simulink model "VDSE_2019b"  (R2025b)
settings: Solver=ode5  StartTime=0.0  StopTime=inf  FixedStep=simulation_step_time  RelTol=1e-3
values from neighbouring files (symbols this model uses):
  A = 1    [vehicle_parameters_script.m]
  bump_height = 0    [vehicle_parameters_script.m]
  bump_length = 1    [vehicle_parameters_script.m]
  bump_time = 1    [vehicle_parameters_script.m]
  cd = 1.8    [vehicle_parameters_script.m]
  cF = 1000    [vehicle_parameters_script.m]
  clF = -cl*(1-Aero_balance)    (= 1.344)    [vehicle_parameters_script.m]
  clR = -cl*Aero_balance    (= 1.456)    [vehicle_parameters_script.m]
  cp_FA = 30    [vehicle_parameters_script.m]
  cp_RA = 13    [vehicle_parameters_script.m]
  cR = 1000    [vehicle_parameters_script.m]
  ctF = tireF.VERTICAL_DAMPING    [vehicle_parameters_script.m]
  ctR = tireR.VERTICAL_DAMPING    [vehicle_parameters_script.m]
  enableAWD = 1    [vehicle_parameters_script.m]
  enableLongDynamics = 1    [vehicle_parameters_script.m]
  enablePowertrain = 1    [vehicle_parameters_script.m]
  Engine_Speed = readmatrix('EngineMap.xlsx','Range','B2:B20')    [vehicle_parameters_script.m]
  Engine_Torque = readmatrix('EngineMap.xlsx','Range','A2:A20')    [vehicle_parameters_script.m]
  exf = 10e-12    (= 1e-11)    [Paceijka52_Parameters.m]
  exr = 10e-12    (= 1e-11)    [Paceijka52_Parameters.m]
  eyf = 1e-12    [Paceijka52_Parameters.m]
  eyr = 1e-12    [Paceijka52_Parameters.m]
  FNOMINf = tireF.FNOMIN    [Paceijka52_Parameters.m]
  FNOMINr = tireR.FNOMIN    [Paceijka52_Parameters.m]
  g = 9.806    [vehicle_parameters_script.m]
  GR = 5.3    [vehicle_parameters_script.m]
  hcog = 0.3054    [vehicle_parameters_script.m]
  hpc = 0.0    (= 0)    [vehicle_parameters_script.m]
  hrcF = 0    [vehicle_parameters_script.m]
  hrcg = (hrcF*lR+hrcR*lF)/(lF+lR)    (= 0)    [vehicle_parameters_script.m]
  hrcR = 0    [vehicle_parameters_script.m]
  huFcog = 0.3054    [vehicle_parameters_script.m]
  huRcog = 0.3054    [vehicle_parameters_script.m]
  JwF = 0.32    [vehicle_parameters_script.m]
  JwR = 0.32    [vehicle_parameters_script.m]
  Jx = 73    [vehicle_parameters_script.m]
  Jy = 230    [vehicle_parameters_script.m]
  Jz = 220    [vehicle_parameters_script.m]
  kF = 40000    [vehicle_parameters_script.m]
  kR = 35000    [vehicle_parameters_script.m]
  kRF = 0    [vehicle_parameters_script.m]
  kRR = 0    [vehicle_parameters_script.m]
  ktF = tireF.VERTICAL_STIFFNESS    [vehicle_parameters_script.m]
  ktR = tireR.VERTICAL_STIFFNESS    [vehicle_parameters_script.m]
  lF = 1.223    [vehicle_parameters_script.m]
  lR = l-lF    (= 0.307)    [vehicle_parameters_script.m]
  m = 258.612    [vehicle_parameters_script.m]
  max_pressure = 1000    [vehicle_parameters_script.m]
  mF = 10.347    [vehicle_parameters_script.m]
  mR = 10.347    [vehicle_parameters_script.m]
  PCX1f = tireF.PCX1    [Paceijka52_Parameters.m]
  PCX1r = tireR.PCX1    [Paceijka52_Parameters.m]
  PCY1f = tireF.PCY1    [Paceijka52_Parameters.m]
  PCY1r = tireR.PCY1    [Paceijka52_Parameters.m]
  PDX1f = tireF.PDX1    [Paceijka52_Parameters.m]
  PDX1r = tireR.PDX1    [Paceijka52_Parameters.m]
  PDX2f = tireF.PDX2    [Paceijka52_Parameters.m]
  PDX2r = tireR.PDX2    [Paceijka52_Parameters.m]
  PDY1f = tireF.PDY1    [Paceijka52_Parameters.m]
  PDY1r = tireR.PDY1    [Paceijka52_Parameters.m]
  PDY2f = tireF.PDY2    [Paceijka52_Parameters.m]
  PDY2r = tireR.PDY2    [Paceijka52_Parameters.m]
  PDY3f = tireF.PDY3    [Paceijka52_Parameters.m]
  PDY3r = tireR.PDY3    [Paceijka52_Parameters.m]
  PEX1f = tireF.PEX1    [Paceijka52_Parameters.m]
  PEX1r = tireR.PEX1    [Paceijka52_Parameters.m]
  PEX2f = tireF.PEX2    [Paceijka52_Parameters.m]
  PEX2r = tireR.PEX2    [Paceijka52_Parameters.m]
  PEX3f = tireF.PEX3    [Paceijka52_Parameters.m]
  PEX3r = tireR.PEX3    [Paceijka52_Parameters.m]
  PEX4f = tireF.PEX4    [Paceijka52_Parameters.m]
  PEX4r = tireR.PEX4    [Paceijka52_Parameters.m]
  PEY1f = tireF.PEY1    [Paceijka52_Parameters.m]
  PEY1r = tireR.PEY1    [Paceijka52_Parameters.m]
  PEY2f = tireF.PEY2    [Paceijka52_Parameters.m]
  PEY2r = tireR.PEY2    [Paceijka52_Parameters.m]
  PEY3f = tireF.PEY3    [Paceijka52_Parameters.m]
  PEY3r = tireR.PEY3    [Paceijka52_Parameters.m]
  PEY4f = tireF.PEY4    [Paceijka52_Parameters.m]
  PEY4r = tireR.PEY4    [Paceijka52_Parameters.m]
  phi0 = 0    [vehicle_parameters_script.m]
  phi_dot0 = 0    [vehicle_parameters_script.m]
  PHX1f = tireF.PHX1    [Paceijka52_Parameters.m]
  PHX1r = tireR.PHX1    [Paceijka52_Parameters.m]
  PHX2f = tireF.PHX2    [Paceijka52_Parameters.m]
  PHX2r = tireR.PHX2    [Paceijka52_Parameters.m]
  PHY1f = tireF.PHY1    [Paceijka52_Parameters.m]
  PHY1r = tireR.PHY1    [Paceijka52_Parameters.m]
  PHY2f = tireF.PHY2    [Paceijka52_Parameters.m]
  PHY2r = tireR.PHY2    [Paceijka52_Parameters.m]
  PHY3f = tireF.PHY3    [Paceijka52_Parameters.m]
  PHY3r = tireR.PHY3    [Paceijka52_Parameters.m]
  PKX1f = tireF.PKX1    [Paceijka52_Parameters.m]
  PKX1r = tireR.PKX1    [Paceijka52_Parameters.m]
  PKX2f = tireF.PKX2    [Paceijka52_Parameters.m]
  PKX2r = tireR.PKX2    [Paceijka52_Parameters.m]
  PKX3f = tireF.PKX3    [Paceijka52_Parameters.m]
  PKX3r = tireR.PKX3    [Paceijka52_Parameters.m]
  PKY1f = tireF.PKY1    [Paceijka52_Parameters.m]
  PKY1r = tireR.PKY1    [Paceijka52_Parameters.m]
  PKY2f = tireF.PKY2    [Paceijka52_Parameters.m]
  PKY2r = tireR.PKY2    [Paceijka52_Parameters.m]
  PKY3f = tireF.PKY3    [Paceijka52_Parameters.m]
  PKY3r = tireR.PKY3    [Paceijka52_Parameters.m]
  psi0 = 0    [vehicle_parameters_script.m]
  psi_dot0 = 0    [vehicle_parameters_script.m]
  PVX1f = tireF.PVX1    [Paceijka52_Parameters.m]
  PVX1r = tireR.PVX1    [Paceijka52_Parameters.m]
  PVX2f = tireF.PVX2    [Paceijka52_Parameters.m]
  PVX2r = tireR.PVX2    [Paceijka52_Parameters.m]
  PVY1f = tireF.PVY1    [Paceijka52_Parameters.m]
  PVY1r = tireR.PVY1    [Paceijka52_Parameters.m]
  PVY2f = tireF.PVY2    [Paceijka52_Parameters.m]
  PVY2r = tireR.PVY2    [Paceijka52_Parameters.m]
  PVY3f = tireF.PVY3    [Paceijka52_Parameters.m]
  PVY3r = tireR.PVY3    [Paceijka52_Parameters.m]
  PVY4f = tireF.PVY4    [Paceijka52_Parameters.m]
  PVY4r = tireR.PVY4    [Paceijka52_Parameters.m]
  QBZ10f = tireF.QBZ10    [Paceijka52_Parameters.m]
  QBZ10r = tireR.QBZ10    [Paceijka52_Parameters.m]
  ... (+143 more)
undefined symbols (not defined in the file or in its folder): Bxf, Bxr, Byf, Byr, Cxf, Cxr, Cyf, Cyr, Dxf, Dxr, Dyf, Dyr, FFB_Gain
libraries: mfeval_LIB x4, sim3dlib x1, sim3dautolib x1, sl3dlib x1
(part 3 of 5)

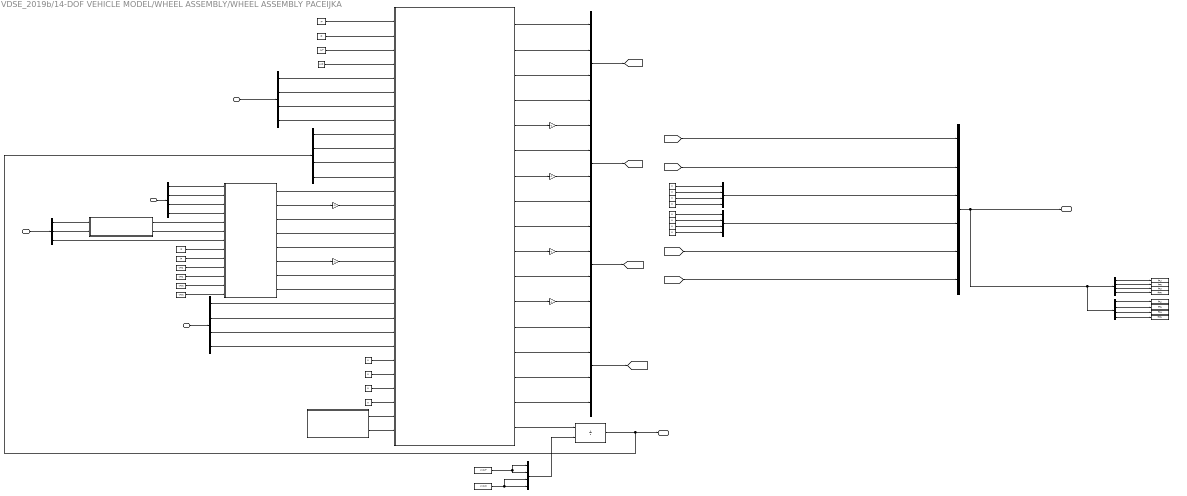
== system VDSE_2019b/14-DOF VEHICLE MODEL/WHEEL ASSEMBLY/WHEEL ASSEMBLY PACEIJKA ==
  note: EXPORTING TIRE FORCES AND MOMENTS
  note: SAVING TIRE FORCES
  steer input [rad] : Inport
  sprung mass outputs : Inport  Port=2
  unsprung masses outputs : Inport  Port=3
  Torques [Nm] : Inport  Port=4
  Bus Creator : BusCreator  Inputs=6
  Bus Creator{1..4,7..8} (6 alike) : BusCreator  Inputs=4
  Bus Selector : BusSelector  OutputSignals=Unsprung masses z Forces [N].FLz_Overall [N],Unsprung masses z Forces [N].FRz_Overall [N],Unsprung masses z Forces [N].RLz_Overall [N],Unsprung masses z Forces [N].RRz_Overall [N]
  Bus Selector2 : BusSelector  OutputSignals=Longitudinal Dynamics.Vx [m/s],Lateral Dynamics.Vy [m/s],Yaw dynamics.psi_dot [rad/s]
  Bus Selector3 : BusSelector  OutputSignals=Steering.deltaFL [rad],Steering.deltaFR [rad],Steering.deltaRL [rad],Steering.deltaRR [rad]
  Bus Selector5 : BusSelector  OutputSignals=TFL [Nm],TFR [Nm],TRL [Nm],TRR [Nm]
  Bus Selector6 : BusSelector  OutputSignals=Tyre x Forces [N].fFLx [N],Tyre x Forces [N].fFRx [N],Tyre x Forces [N].fRLx [N],Tyre x Forces [N].fRRx [N]
  Bus Selector7 : BusSelector  OutputSignals=Tyre y Forces [N].fFLy [N],Tyre y Forces [N].fFRy [N],Tyre y Forces [N].fRLy [N],Tyre y Forces [N].fRRy [N]
  Constant{,26..28} (4 alike) : Constant  Value=0
  Constant1 : Constant  Value=wF/2
  Constant13 : Constant  Value=lF
  Constant14 : Constant  Value=lR
  Constant2 : Constant  Value=wF/2
  Constant20 : Constant  Value=rF
  Constant21 : Constant  Value=rR
  Constant22 : Constant  Value=JwF
  Constant23 : Constant  Value=JwR
  Constant24 : Constant  Value=Vx0/rF
  Constant25 : Constant  Value=Vx0/rR
  Constant3 : Constant  Value=wR/2
  Constant4 : Constant  Value=wR/2
  Demux1 : Demux
  Gain{,1..5} (6 alike) : Gain  Gain=-1
  Integrator1 : Integrator  InitialConditionSource=external
  Mux2 : Mux
  SIDE SLIP ANGLE CALCULATION : Subsystem
  TIRE FORCES AND WHEEL DYNAMICS : MATLAB Function  TreatAsAtomicUnit=on
  TIRE PARAMETERS : Subsystem
  TIRE VELOCITIES : MATLAB Function  TreatAsAtomicUnit=on
  To Workspace : ToWorkspace  VariableName=fFLx  SaveFormat=Timeseries  SampleTime=-1
  To Workspace1 : ToWorkspace  VariableName=fFRx  SaveFormat=Timeseries  SampleTime=-1
  To Workspace2 : ToWorkspace  VariableName=fRLx  SaveFormat=Timeseries  SampleTime=-1
  To Workspace3 : ToWorkspace  VariableName=fRRx  SaveFormat=Timeseries  SampleTime=-1
  To Workspace4 : ToWorkspace  VariableName=fFLy  SaveFormat=Timeseries  SampleTime=-1
  To Workspace5 : ToWorkspace  VariableName=fFRy  SaveFormat=Timeseries  SampleTime=-1
  To Workspace6 : ToWorkspace  VariableName=fRLy  SaveFormat=Timeseries  SampleTime=-1
  To Workspace7 : ToWorkspace  VariableName=fRRy  SaveFormat=Timeseries  SampleTime=-1
  Zero{,1..7} (8 alike) : Constant  Value=0  OutDataTypeStr=Inherit: Inherit via back propagation
  Tyre Forces and Moments : Outport
  Wheel Speeds [rad/s] : Outport  Port=2
  wires:
  Zero/1 -> Bus Creator3/1  "fFLz [N]"
  Zero2/1 -> Bus Creator3/3  "fRLz [N]"
  Zero4/1 -> Bus Creator4/1  "mFLx [Nm]"
  Zero1/1 -> Bus Creator3/2  "fFRz [N]"
  Zero7/1 -> Bus Creator4/4  "mRRx [Nm]"
  Zero5/1 -> Bus Creator4/2  "mFRx [Nm]"
  Zero3/1 -> Bus Creator3/4  "fRRz [N]"
  Zero6/1 -> Bus Creator4/3  "mRLx [Nm]"
  Bus Creator2/1 -> [Tyre_y_Forces]  "Tyre y Forces [N]"
  TIRE FORCES AND WHEEL DYNAMICS/7(fRLy) -> Gain2/1  "fRLy [N]"
  TIRE FORCES AND WHEEL DYNAMICS/5(fFLy) -> Gain3/1  "fFLy [N]"
  Bus Creator1/1 -> [Tyre_x_Forces]  "Tyre x Forces [N]"
  TIRE VELOCITIES/8(VRRy) -> TIRE FORCES AND WHEEL DYNAMICS/20(VRRy)  "VRRy"
  TIRE VELOCITIES/7(VRRx) -> TIRE FORCES AND WHEEL DYNAMICS/19(VRRx)  "VRRx"
  Integrator1/1 -> Wheel Speeds [rad/s]/1, Demux1/1  "omega [rad/s]"
  Demux1/4 -> TIRE FORCES AND WHEEL DYNAMICS/12(omegaRR)
  Demux1/3 -> TIRE FORCES AND WHEEL DYNAMICS/11(omegaRL)
  Demux1/2 -> TIRE FORCES AND WHEEL DYNAMICS/10(omegaFR)
  Demux1/1 -> TIRE FORCES AND WHEEL DYNAMICS/9(omegaFL)
  TIRE FORCES AND WHEEL DYNAMICS/17(omega_dot) -> Integrator1/1  "omegas_dot [rad/s^2]"
  Constant25/1 -> Mux2/4, Mux2/3
  Mux2/1 -> Integrator1/2
  Constant24/1 -> Mux2/1, Mux2/2
  Constant21/1 -> TIRE FORCES AND WHEEL DYNAMICS/2(rR)
  Constant23/1 -> TIRE FORCES AND WHEEL DYNAMICS/4(JwR)
  Constant22/1 -> TIRE FORCES AND WHEEL DYNAMICS/3(JwF)
  Constant20/1 -> TIRE FORCES AND WHEEL DYNAMICS/1(rF)
  TIRE VELOCITIES/2(VFLy) -> Gain/1  "VFLy"
  TIRE VELOCITIES/1(VFLx) -> TIRE FORCES AND WHEEL DYNAMICS/13(VFLx)  "VFLx"
  TIRE VELOCITIES/4(VFRy) -> TIRE FORCES AND WHEEL DYNAMICS/16(VFRy)  "VFRy"
  Constant4/1 -> TIRE VELOCITIES/13(wRR)
  Constant13/1 -> TIRE VELOCITIES/8(lF)
  Constant1/1 -> TIRE VELOCITIES/10(wFL)
  Constant14/1 -> TIRE VELOCITIES/9(lR)
  Constant2/1 -> TIRE VELOCITIES/11(wFR)
  TIRE VELOCITIES/5(VRLx) -> TIRE FORCES AND WHEEL DYNAMICS/17(VRLx)  "VRLx"
  Constant3/1 -> TIRE VELOCITIES/12(wRL)
  TIRE VELOCITIES/3(VFRx) -> TIRE FORCES AND WHEEL DYNAMICS/15(VFRx)  "VFRx"
  TIRE VELOCITIES/6(VRLy) -> Gain1/1  "VRLy"
  SIDE SLIP ANGLE CALCULATION/2(beta [rad]) -> TIRE VELOCITIES/6(beta)  "beta"
  SIDE SLIP ANGLE CALCULATION/1(V [m/s]) -> TIRE VELOCITIES/5(V)  "V"
  Bus Selector/1 -> TIRE FORCES AND WHEEL DYNAMICS/5(fFLz)  "<FLz_Overall [N]>"
  Bus Selector/4 -> TIRE FORCES AND WHEEL DYNAMICS/8(fRRz)  "<RRz_Overall [N]>"
  Bus Selector/3 -> TIRE FORCES AND WHEEL DYNAMICS/7(fRLz)  "<RLz_Overall [N]>"
  Bus Selector/2 -> TIRE FORCES AND WHEEL DYNAMICS/6(fFRz)  "<FRz_Overall [N]>"
  unsprung masses outputs/1 -> Bus Selector/1
  sprung mass outputs/1 -> Bus Selector2/1
  Bus Selector3/2 -> TIRE VELOCITIES/2(deltaFR)  "<deltaFR [rad]>"
  Bus Selector3/4 -> TIRE VELOCITIES/4(deltaRR)  "<deltaRR [rad]>"
  Bus Selector3/1 -> TIRE VELOCITIES/1(deltaFL)  "<deltaFL [rad]>"
  Bus Selector3/3 -> TIRE VELOCITIES/3(deltaRL)  "<deltaRL [rad]>"
  steer input [rad]/1 -> Bus Selector3/1
  Bus Creator/1 -> Bus Selector7/1, Bus Selector6/1, Tyre Forces and Moments/1
  Torques [Nm]/1 -> Bus Selector5/1
  Bus Selector6/1 -> To Workspace/1  "<fFLx [N]>"
  Bus Selector6/2 -> To Workspace1/1  "<fFRx [N]>"
  Bus Selector6/3 -> To Workspace2/1  "<fRLx [N]>"
  Bus Selector6/4 -> To Workspace3/1  "<fRRx [N]>"
  Bus Selector7/1 -> To Workspace4/1  "<fFLy [N]>"
  Bus Selector7/2 -> To Workspace5/1  "<fFRy [N]>"
  Bus Selector7/3 -> To Workspace6/1  "<fRLy [N]>"
  Bus Selector7/4 -> To Workspace7/1  "<fRRy [N]>"
  [Tyre_y_Moments] -> Bus Creator/5  "Tyre My Moments [Nm]"
  Constant/1 -> TIRE FORCES AND WHEEL DYNAMICS/25(gammaFL)
  Constant26/1 -> TIRE FORCES AND WHEEL DYNAMICS/26(gammaFR)
  Constant27/1 -> TIRE FORCES AND WHEEL DYNAMICS/27(gammaRL)
  Constant28/1 -> TIRE FORCES AND WHEEL DYNAMICS/28(gammaRR)
  TIRE PARAMETERS/1(Tire Parameters Front Axle) -> TIRE FORCES AND WHEEL DYNAMICS/29(TireParams_front)
  TIRE PARAMETERS/2(Tire Parameters Rear Axle) -> TIRE FORCES AND WHEEL DYNAMICS/30(TireParams_rear)
  Gain/1 -> TIRE FORCES AND WHEEL DYNAMICS/14(VFLy)  "VFLy"
  Gain1/1 -> TIRE FORCES AND WHEEL DYNAMICS/18(VRLy)  "VRLy"
  TIRE FORCES AND WHEEL DYNAMICS/1(fFLx) -> Bus Creator1/1  "fFLx [N]"
  TIRE FORCES AND WHEEL DYNAMICS/2(fFRx) -> Bus Creator1/2  "fFRx [N]"
  TIRE FORCES AND WHEEL DYNAMICS/3(fRLx) -> Bus Creator1/3  "fRLx [N]"
  TIRE FORCES AND WHEEL DYNAMICS/4(fRRx) -> Bus Creator1/4  "fRRx [N]"
  Gain3/1 -> Bus Creator2/1  "fFLy [N]"
  TIRE FORCES AND WHEEL DYNAMICS/6(fFRy) -> Bus Creator2/2  "fFRy [N]"
  Gain2/1 -> Bus Creator2/3  "fRLy [N]"
  TIRE FORCES AND WHEEL DYNAMICS/8(fRRy) -> Bus Creator2/4  "fRRy [N]"
  [Tyre_x_Forces] -> Bus Creator/1  "Tyre x Forces [N]"
  [Tyre_y_Forces] -> Bus Creator/2  "Tyre y Forces [N]"
  Bus Creator3/1 -> Bus Creator/3  "Tyre z Forces [N]"
  Bus Creator4/1 -> Bus Creator/4  "Tyre Mx Moments [Nm]"
  [Tyre_z_Moments] -> Bus Creator/6  "Tyre Mz Moments [Nm]"
  TIRE FORCES AND WHEEL DYNAMICS/9(mFLz) -> Bus Creator7/1  "mFLz [Nm]"
  TIRE FORCES AND WHEEL DYNAMICS/10(mFRz) -> Gain4/1  "mFRz [Nm]"
  Gain4/1 -> Bus Creator7/2  "mFRz [Nm]"
  TIRE FORCES AND WHEEL DYNAMICS/11(mRLz) -> Bus Creator7/3  "mRLz [Nm]"
  TIRE FORCES AND WHEEL DYNAMICS/12(mRRz) -> Gain5/1  "mRRz [Nm]"
  Gain5/1 -> Bus Creator7/4  "mRRz [Nm]"
  TIRE FORCES AND WHEEL DYNAMICS/13(mFLy) -> Bus Creator8/1  "mFLy [Nm]"
  TIRE FORCES AND WHEEL DYNAMICS/14(mFRy) -> Bus Creator8/2  "mFRy [Nm]"
  TIRE FORCES AND WHEEL DYNAMICS/15(mRLy) -> Bus Creator8/3  "mRLy [Nm]"
  TIRE FORCES AND WHEEL DYNAMICS/16(mRRy) -> Bus Creator8/4  "mRRy [Nm]"
  Bus Creator7/1 -> [Tyre_z_Moments]  "Tyre Mz Moments [Nm]"
  Bus Creator8/1 -> [Tyre_y_Moments]  "Tyre My Moments [Nm]"
  Bus Selector2/1 -> SIDE SLIP ANGLE CALCULATION/1(Vx [m/s])  "<Vx [m/s]>"
  Bus Selector2/2 -> SIDE SLIP ANGLE CALCULATION/2(Vy [m/s])  "<Vy [m/s]>"
  Bus Selector2/3 -> TIRE VELOCITIES/7(psidot)  "<psi_dot [rad/s]>"
  Bus Selector5/1 -> TIRE FORCES AND WHEEL DYNAMICS/21(TFL)  "<TFL [Nm]>"
  Bus Selector5/2 -> TIRE FORCES AND WHEEL DYNAMICS/22(TFR)  "<TFR [Nm]>"
  Bus Selector5/3 -> TIRE FORCES AND WHEEL DYNAMICS/23(TRL)  "<TRL [Nm]>"
  Bus Selector5/4 -> TIRE FORCES AND WHEEL DYNAMICS/24(TRR)  "<TRR [Nm]>"

== system VDSE_2019b/14-DOF VEHICLE MODEL/EQUATIONS OF MOTION FOR CHASSIS/Pitch Dynamics/Downforce ==
  Vx : Inport
  Gain : Gain  Gain=-0.5*rho*clF*A
  Gain{1,3,5,7} (4 alike) : Gain  Gain=0.5
  Gain2 : Gain  Gain=-0.5*rho*clF*A
  Gain4 : Gain  Gain=-0.5*rho*clR*A
  Gain6 : Gain  Gain=-0.5*rho*clR*A
  Square{,1..3} (4 alike) : Math  Operator=square
  fFLz_overall : Outport
  fFRz_overall : Outport  Port=2
  fRLz_overall : Outport  Port=3
  fRRz_overall : Outport  Port=4
  wires:
  Gain/1 -> Gain1/1
  Square/1 -> Gain/1
  Gain1/1 -> fFLz_overall/1
  Square1/1 -> Gain2/1
  Gain2/1 -> Gain3/1
  Gain3/1 -> fFRz_overall/1
  Vx/1 -> Square/1, Square1/1, Square2/1, Square3/1
  Gain6/1 -> Gain7/1
  Square3/1 -> Gain6/1
  Square2/1 -> Gain4/1
  Gain4/1 -> Gain5/1
  Gain5/1 -> fRLz_overall/1
  Gain7/1 -> fRRz_overall/1

== system VDSE_2019b/14-DOF VEHICLE MODEL/EQUATIONS OF MOTION FOR CHASSIS/Roll Dynamics/Downforce ==
  Vx : Inport
  Gain : Gain  Gain=-0.5*rho*clF*A
  Gain{1,3,5,7} (4 alike) : Gain  Gain=0.5
  Gain2 : Gain  Gain=-0.5*rho*clF*A
  Gain4 : Gain  Gain=-0.5*rho*clR*A
  Gain6 : Gain  Gain=-0.5*rho*clR*A
  Square{,1..3} (4 alike) : Math  Operator=square
  fFLz_overall : Outport
  fFRz_overall : Outport  Port=2
  fRLz_overall : Outport  Port=3
  fRRz_overall : Outport  Port=4
  wires:
  Gain/1 -> Gain1/1
  Square/1 -> Gain/1
  Gain1/1 -> fFLz_overall/1
  Square1/1 -> Gain2/1
  Gain2/1 -> Gain3/1
  Gain3/1 -> fFRz_overall/1
  Vx/1 -> Square/1, Square1/1, Square2/1, Square3/1
  Gain6/1 -> Gain7/1
  Square3/1 -> Gain6/1
  Square2/1 -> Gain4/1
  Gain4/1 -> Gain5/1
  Gain5/1 -> fRLz_overall/1
  Gain7/1 -> fRRz_overall/1

== system VDSE_2019b/14-DOF VEHICLE MODEL/EQUATIONS OF MOTION FOR CHASSIS/Vertical Dynamics/Downforce ==
  Vx : Inport
  Gain : Gain  Gain=-0.5*rho*clF*A
  Gain{1,3,5,7} (4 alike) : Gain  Gain=0.5
  Gain2 : Gain  Gain=-0.5*rho*clF*A
  Gain4 : Gain  Gain=-0.5*rho*clR*A
  Gain6 : Gain  Gain=-0.5*rho*clR*A
  Square{,1..3} (4 alike) : Math  Operator=square
  fFLz_overall : Outport
  fFRz_overall : Outport  Port=2
  fRLz_overall : Outport  Port=3
  fRRz_overall : Outport  Port=4
  wires:
  Gain/1 -> Gain1/1
  Square/1 -> Gain/1
  Gain1/1 -> fFLz_overall/1
  Square1/1 -> Gain2/1
  Gain2/1 -> Gain3/1
  Gain3/1 -> fFRz_overall/1
  Vx/1 -> Square/1, Square1/1, Square2/1, Square3/1
  Gain6/1 -> Gain7/1
  Square3/1 -> Gain6/1
  Square2/1 -> Gain4/1
  Gain4/1 -> Gain5/1
  Gain5/1 -> fRLz_overall/1
  Gain7/1 -> fRRz_overall/1

== system VDSE_2019b/14-DOF VEHICLE MODEL/SUSPENSION/FRONT SUSPENSION/SUSPENSION FL ==
  z [m] : Inport
  Vz [m/s] : Inport  Port=2
  phi [rad] : Inport  Port=3
  phi_dot [rad/s] : Inport  Port=4
  theta [rad] : Inport  Port=5
  theta_dot [rad/s] : Inport  Port=6
  zFR [m] : Inport  Port=7
  yFL_road [m] : Inport  Port=8
  FL : Subsystem
  TIRE VERTICAL DEFLECTION : Subsystem
  fFLz [N] : Outport
  zFL_dot [m/s] : Outport  Port=2
  zFL [m] : Outport  Port=3
  wires:
  FL/2(zFL_dot [m/s]) -> TIRE VERTICAL DEFLECTION/2(zFL_dot [m/s]), zFL_dot [m/s]/1
  z [m]/1 -> FL/1(z [m])
  TIRE VERTICAL DEFLECTION/1(fFLz [N]) -> fFLz [N]/1
  theta [rad]/1 -> FL/5(theta [rad])
  zFR [m]/1 -> FL/7(zFR [m])
  Vz [m/s]/1 -> FL/2(Vz [m/s])
  yFL_road [m]/1 -> TIRE VERTICAL DEFLECTION/3(yFL_road [m]), FL/8(yFL_road [m])
  phi_dot [rad/s]/1 -> FL/4(phi_dot [rad/s])
  FL/1(zFL [m]) -> TIRE VERTICAL DEFLECTION/1(zFL [m]), zFL [m]/1
  phi [rad]/1 -> FL/3(phi [rad])
  theta_dot [rad/s]/1 -> FL/6(theta_dot [rad/s])

== system VDSE_2019b/14-DOF VEHICLE MODEL/SUSPENSION/FRONT SUSPENSION/SUSPENSION FR ==
  z [m] : Inport
  Vz [m/s] : Inport  Port=2
  phi [rad] : Inport  Port=3
  phi_dot [rad/s] : Inport  Port=4
  theta [rad] : Inport  Port=5
  theta_dot [rad/s] : Inport  Port=6
  zFL [m] : Inport  Port=7
  yFR_road [m] : Inport  Port=8
  FR : Subsystem
  TIRE VERTICAL DEFLECTION : Subsystem
  fFRz [N] : Outport
  zFR [m] : Outport  Port=2
  zFR_dot [m/s] : Outport  Port=3
  wires:
  FR/2(zFR_dot [m/s]) -> zFR_dot [m/s]/1, TIRE VERTICAL DEFLECTION/2(zFR_dot [m/s])
  yFR_road [m]/1 -> FR/8(yFR_road [m]), TIRE VERTICAL DEFLECTION/3(yFR_road [m])
  z [m]/1 -> FR/1(z [m])
  TIRE VERTICAL DEFLECTION/1(fFRz [N]) -> fFRz [N]/1
  theta [rad]/1 -> FR/5(theta [rad])
  zFL [m]/1 -> FR/7(zFL [m])
  Vz [m/s]/1 -> FR/2(Vz [m/s])
  phi_dot [rad/s]/1 -> FR/4(phi_dot [rad/s])
  FR/1(zFR [m]) -> TIRE VERTICAL DEFLECTION/1(zFR [m]), zFR [m]/1
  phi [rad]/1 -> FR/3(phi [rad])
  theta_dot [rad/s]/1 -> FR/6(theta_dot [rad/s])

== system VDSE_2019b/14-DOF VEHICLE MODEL/SUSPENSION/Load Transfer/Coupling of load transfer and suspension reaction ==
  Longidutinal Load Transfer [N] : Inport
  Lateral Load Transfer - Front [N] : Inport  Port=2
  Lateral Load Transfer - Rear [N] : Inport  Port=3
  <fFLz [N]> : Inport  Port=4
  <fFRz [N]> : Inport  Port=5
  <fRLz [N]> : Inport  Port=6
  <fRRz [N]> : Inport  Port=7
  Add{,1..4} (5 alike) : Sum
  Add5 : Sum  Inputs=+-
  Add6 : Sum  Inputs=-+
  Add7 : Sum  Inputs=--
  Lateral Load Transfer - Front [N]1 : InportShadow  Port=2
  Lateral Load Transfer - Rear [N]1 : InportShadow  Port=3
  Longidutinal Load Transfer [N]1 : InportShadow
  Longidutinal Load Transfer [N]2 : InportShadow
  Longidutinal Load Transfer [N]3 : InportShadow
  FLz_Overall [N] : Outport
  FRz_Overall [N] : Outport  Port=2
  RLz_Overall [N] : Outport  Port=3
  RRz_Overall [N] : Outport  Port=4
  wires:
  <fFRz [N]>/1 -> Add1/2
  Lateral Load Transfer - Rear [N]/1 -> Add5/2
  Longidutinal Load Transfer [N]/1 -> Add7/1
  Add7/1 -> Add/1  "FL Dynamic LT"
  Lateral Load Transfer - Front [N]/1 -> Add7/2
  Add4/1 -> Add3/1  "RR Dynamic LT"
  Add6/1 -> Add1/1  "FR Dynamic LT"
  Add5/1 -> Add2/1  "RL Dynamic LT"
  <fRRz [N]>/1 -> Add3/2
  <fFLz [N]>/1 -> Add/2
  <fRLz [N]>/1 -> Add2/2
  Add1/1 -> FRz_Overall [N]/1  "FRz_Overall [N]"
  Add3/1 -> RRz_Overall [N]/1  "RRz_Overall [N]"
  Add/1 -> FLz_Overall [N]/1  "FLz_Overall [N]"
  Add2/1 -> RLz_Overall [N]/1  "RLz_Overall [N]"
  Longidutinal Load Transfer [N]1/1 -> Add6/1
  Longidutinal Load Transfer [N]2/1 -> Add5/1
  Longidutinal Load Transfer [N]3/1 -> Add4/1
  Lateral Load Transfer - Front [N]1/1 -> Add6/2
  Lateral Load Transfer - Rear [N]1/1 -> Add4/2

== system VDSE_2019b/14-DOF VEHICLE MODEL/SUSPENSION/Load Transfer/Dynamic Lateral Load Transfer - Front ==
  ay [m/s^2] : Inport
  Add : Sum
  Gain : Gain  Gain=lR/(lR+lF)
  Gain1 : Gain  Gain=2*mF*huFcog/wF
  Gain2 : Gain  Gain=m*hrcF/wF
  Lat. Dynamic Transfer [N] : Outport
  wires:
  ay [m/s^2]/1 -> Gain2/1, Gain1/1
  Gain2/1 -> Gain/1
  Add/1 -> Lat. Dynamic Transfer [N]/1
  Gain1/1 -> Add/2
  Gain/1 -> Add/1

== system VDSE_2019b/14-DOF VEHICLE MODEL/SUSPENSION/Load Transfer/Dynamic Lateral Load Transfer - Rear ==
  ay [m/s^2] : Inport
  Add : Sum
  Gain : Gain  Gain=lF/(lR+lF)
  Gain1 : Gain  Gain=2*mR*huRcog/wR
  Gain2 : Gain  Gain=m*hrcR/wR
  Lat. Dynamic Transfer [N] : Outport
  wires:
  Add/1 -> Lat. Dynamic Transfer [N]/1
  Gain1/1 -> Add/2
  ay [m/s^2]/1 -> Gain2/1, Gain1/1
  Gain2/1 -> Gain/1
  Gain/1 -> Add/1

== system VDSE_2019b/14-DOF VEHICLE MODEL/SUSPENSION/Load Transfer/Dynamic Longitudinal Load Transfer ==
  ax [m/s^2] : Inport
  Add : Sum
  Gain : Gain  Gain=1/2*hpc*m/(lF+lR)/2
  Gain1 : Gain  Gain=(mF*huFcog + mR*huRcog)/(lF+lR)
  Long. Dynamic Transfer [N] : Outport
  wires:
  ax [m/s^2]/1 -> Gain1/1, Gain/1
  Gain/1 -> Add/1
  Add/1 -> Long. Dynamic Transfer [N]/1
  Gain1/1 -> Add/2

== system VDSE_2019b/14-DOF VEHICLE MODEL/SUSPENSION/REAR SUSPENSION/SUSPENSION RL ==
  z [m] : Inport
  Vz [m/s] : Inport  Port=2
  phi [rad] : Inport  Port=3
  phi_dot [rad/s] : Inport  Port=4
  theta [rad] : Inport  Port=5
  theta_dot [rad/s] : Inport  Port=6
  zRR [m] : Inport  Port=7
  yRL_road [m] : Inport  Port=8
  RL : Subsystem
  TIRE VERTICAL DEFLECTION : Subsystem
  fRLz [N] : Outport
  zRL_dot [m/s] : Outport  Port=2
  zRL [m] : Outport  Port=3
  wires:
  RL/2(zRL_dot [m/s]) -> TIRE VERTICAL DEFLECTION/2(zRL_dot [m/s]), zRL_dot [m/s]/1
  z [m]/1 -> RL/1(z [m])
  TIRE VERTICAL DEFLECTION/1(fRLz [N]) -> fRLz [N]/1  "fRLz [N]"
  theta [rad]/1 -> RL/5(theta [rad])
  zRR [m]/1 -> RL/7(zRR [m])
  Vz [m/s]/1 -> RL/2(Vz [m/s])
  yRL_road [m]/1 -> TIRE VERTICAL DEFLECTION/3(yRL_road [m]), RL/8(yRL_road [m])
  phi_dot [rad/s]/1 -> RL/4(phi_dot [rad/s])
  RL/1(zRL [m]) -> TIRE VERTICAL DEFLECTION/1(zRL [m]), zRL [m]/1
  phi [rad]/1 -> RL/3(phi [rad])
  theta_dot [rad/s]/1 -> RL/6(theta_dot [rad/s])

== system VDSE_2019b/14-DOF VEHICLE MODEL/SUSPENSION/REAR SUSPENSION/SUSPENSION RR ==
  z [m] : Inport
  Vz [m/s] : Inport  Port=2
  phi [rad] : Inport  Port=3
  phi_dot [rad/s] : Inport  Port=4
  theta [rad] : Inport  Port=5
  theta_dot [rad/s] : Inport  Port=6
  zRL [m] : Inport  Port=7
  yRR_road [m] : Inport  Port=8
  RR : Subsystem
  TIRE VERTICAL DEFLECTION : Subsystem
  fRRz [N] : Outport
  zRR [m] : Outport  Port=2
  zRR_dot [m/s] : Outport  Port=3
  wires:
  RR/2(zRR_dot [m/s]) -> TIRE VERTICAL DEFLECTION/2(zRR_dot [m/s]), zRR_dot [m/s]/1
  yRR_road [m]/1 -> TIRE VERTICAL DEFLECTION/3(yRR_road [m]), RR/8(yRR_road [m])
  z [m]/1 -> RR/1(z [m])
  TIRE VERTICAL DEFLECTION/1(fRRz [N]) -> fRRz [N]/1
  theta [rad]/1 -> RR/5(theta [rad])
  zRL [m]/1 -> RR/7(zRL [m])
  Vz [m/s]/1 -> RR/2(Vz [m/s])
  phi_dot [rad/s]/1 -> RR/4(phi_dot [rad/s])
  RR/1(zRR [m]) -> TIRE VERTICAL DEFLECTION/1(zRR [m]), zRR [m]/1
  phi [rad]/1 -> RR/3(phi [rad])
  theta_dot [rad/s]/1 -> RR/6(theta_dot [rad/s])

== system VDSE_2019b/14-DOF VEHICLE MODEL/WHEEL ASSEMBLY/WHEEL ASSEMBLY BCD/SIDE SLIP ANGLE CALCULATION ==
  Vx [m/s] : Inport
  Vy [m/s] : Inport  Port=2
  Add : Sum
  Atan2 : Trigonometry  Operator=atan2
  Clock : Clock
  Constant : Constant  Value=enableLongDynamics
  Constant1 : Constant  Value=Vx0
  Constant2 : Constant  Value=0
  Sqrt : Sqrt
  Square : Math  Operator=square
  Square1 : Math  Operator=square
  Switch : Switch  Criteria=u2 > Threshold  SaturateOnIntegerOverflow=off  InputSameDT=off
  Switch1 : Switch  Criteria=u2 > Threshold  Threshold=0.01  SaturateOnIntegerOverflow=off  InputSameDT=off
  Vy [m/s]1 : InportShadow  Port=2
  V [m/s] : Outport
  beta [rad] : Outport  Port=2
  wires:
  Clock/1 -> Switch1/2
  Constant2/1 -> Switch1/3
  Switch1/1 -> Switch/2
  Constant1/1 -> Switch/3
  Constant/1 -> Switch1/1
  Switch/1 -> Atan2/2, Square/1
  Square1/1 -> Add/2
  Square/1 -> Add/1
  Vy [m/s]/1 -> Square1/1
  Vx [m/s]/1 -> Switch/1
  Add/1 -> Sqrt/1
  Sqrt/1 -> V [m/s]/1
  Atan2/1 -> beta [rad]/1
  Vy [m/s]1/1 -> Atan2/1

== system VDSE_2019b/14-DOF VEHICLE MODEL/WHEEL ASSEMBLY/WHEEL ASSEMBLY BCD/TIRE PARAMETERS ==
  Constant : Constant  Value=Bxf
  Constant1 : Constant  Value=Cxf
  Constant10 : Constant  Value=Cyr
  Constant11 : Constant  Value=Dyr
  Constant2 : Constant  Value=Dxf
  Constant3 : Constant  Value=Bxr
  Constant4 : Constant  Value=Cxr
  Constant5 : Constant  Value=Dxr
  Constant6 : Constant  Value=Byf
  Constant7 : Constant  Value=Cyf
  Constant8 : Constant  Value=Dyf
  Constant9 : Constant  Value=Byr
  Bxf : Outport
  Cxf : Outport  Port=2
  Dxf : Outport  Port=3
  Bxr : Outport  Port=4
  Cxr : Outport  Port=5
  Dxr : Outport  Port=6
  Byf : Outport  Port=7
  Cyf : Outport  Port=8
  Dyf : Outport  Port=9
  Byr : Outport  Port=10
  Cyr : Outport  Port=11
  Dyr : Outport  Port=12
  wires:
  Constant/1 -> Bxf/1
  Constant1/1 -> Cxf/1
  Constant2/1 -> Dxf/1
  Constant5/1 -> Dxr/1
  Constant4/1 -> Cxr/1
  Constant3/1 -> Bxr/1
  Constant9/1 -> Byr/1
  Constant10/1 -> Cyr/1
  Constant11/1 -> Dyr/1
  Constant8/1 -> Dyf/1
  Constant7/1 -> Cyf/1
  Constant6/1 -> Byf/1

== system VDSE_2019b/14-DOF VEHICLE MODEL/WHEEL ASSEMBLY/WHEEL ASSEMBLY MFEVAL/SIDE SLIP ANGLE CALCULATION ==
  Vx [m/s] : Inport
  Vy [m/s] : Inport  Port=2
  Add : Sum
  Atan2 : Trigonometry  Operator=atan2
  Clock : Clock
  Constant : Constant  Value=enableLongDynamics
  Constant1 : Constant  Value=Vx0
  Constant2 : Constant  Value=0
  Sqrt : Sqrt
  Square : Math  Operator=square
  Square1 : Math  Operator=square
  Switch : Switch  Criteria=u2 > Threshold  SaturateOnIntegerOverflow=off  InputSameDT=off
  Switch1 : Switch  Criteria=u2 > Threshold  Threshold=0.01  SaturateOnIntegerOverflow=off  InputSameDT=off
  Vy [m/s]1 : InportShadow  Port=2
  V [m/s] : Outport
  beta [rad] : Outport  Port=2
  wires:
  Clock/1 -> Switch1/2
  Constant2/1 -> Switch1/3
  Switch1/1 -> Switch/2
  Constant1/1 -> Switch/3
  Constant/1 -> Switch1/1
  Square1/1 -> Add/2
  Square/1 -> Add/1
  Vy [m/s]/1 -> Square1/1
  Vx [m/s]/1 -> Switch/1
  Add/1 -> Sqrt/1
  Atan2/1 -> beta [rad]/1
  Vy [m/s]1/1 -> Atan2/1
  Switch/1 -> Atan2/2, Square/1
  Sqrt/1 -> V [m/s]/1

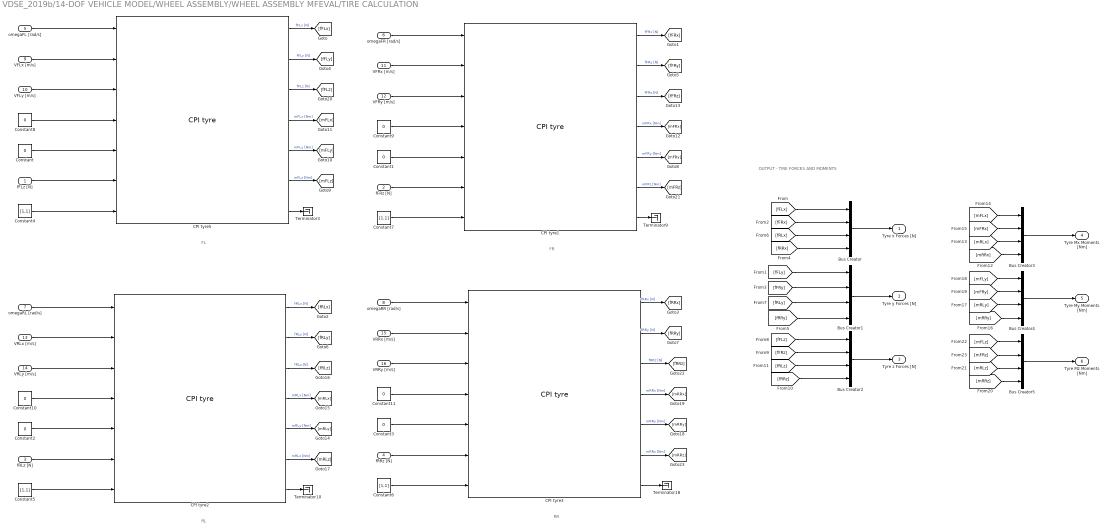
== system VDSE_2019b/14-DOF VEHICLE MODEL/WHEEL ASSEMBLY/WHEEL ASSEMBLY MFEVAL/TIRE CALCULATION ==
  note: RR
  note: RL
  note: FR
  note: FL
  note: OUTPUT - TIRE FORCES AND MOMENTS
  fFLz [N] : Inport
  fFRz [N] : Inport  Port=2
  fRLz [N] : Inport  Port=3
  fRRz [N] : Inport  Port=4
  omegaFL [rad/s] : Inport  Port=5
  omegaFR [rad/s] : Inport  Port=6
  omegaRL [rad/s] : Inport  Port=7
  omegaRR [rad/s] : Inport  Port=8
  VFLx [m/s] : Inport  Port=9
  VFLy [m/s] : Inport  Port=10
  VFRx [m/s] : Inport  Port=11
  VFRy [m/s] : Inport  Port=12
  VRLx [m/s] : Inport  Port=13
  VRLy [m/s] : Inport  Port=14
  VRRx [m/s] : Inport  Port=15
  VRRy [m/s] : Inport  Port=16
  Bus Creator{,1..5} (6 alike) : BusCreator  Inputs=4
  CPI tyre1 : mfeval_LIB/CPI tyre  Description=Magic Formula 6.1.2 tyre model including relaxation length and transient calculations  userParameterSource=tir_file_front  userSide=2 right  userDynamics=1 steady state  userUseMode=1 combined  enablePressure=off  userPressure=2.3
      settings: SourceProductName=MFeval Library
  CPI tyre2 : mfeval_LIB/CPI tyre  Description=Magic Formula 6.1.2 tyre model including relaxation length and transient calculations  userParameterSource=tir_file_rear  userSide=1 left  userDynamics=1 steady state  userUseMode=1 combined  enablePressure=off  userPressure=2.3
      settings: SourceProductName=MFeval Library
  CPI tyre3 : mfeval_LIB/CPI tyre  Description=Magic Formula 6.1.2 tyre model including relaxation length and transient calculations  userParameterSource=tir_file_rear  userSide=2 right  userDynamics=1 steady state  userUseMode=1 combined  enablePressure=off  userPressure=2.3
      settings: SourceProductName=MFeval Library
  CPI tyre5 : mfeval_LIB/CPI tyre  Description=Magic Formula 6.1.2 tyre model including relaxation length and transient calculations  userParameterSource=tir_file_front  userSide=1 left  userDynamics=1 steady state  userUseMode=1 combined  enablePressure=off  userPressure=2.3
      settings: SourceProductName=MFeval Library
  Constant{,1..3,8..11} (8 alike) : Constant  Value=0
  Constant{4..7} (4 alike) : Constant  Value=[1,1]
  Terminator{3,9..10,18} (4 alike) : Terminator
  Tyre x Forces [N] : Outport
  Tyre y Forces [N] : Outport  Port=2
  Tyre z Forces [N] : Outport  Port=3
  Tyre Mx Moments [Nm] : Outport  Port=4
  Tyre My Moments [Nm] : Outport  Port=5
  Tyre Mz Moments [Nm] : Outport  Port=6
  wires:
  Constant11/1 -> CPI tyre3/4
  Constant10/1 -> CPI tyre2/4
  Constant9/1 -> CPI tyre1/4
  Constant8/1 -> CPI tyre5/4
  CPI tyre3/3 -> [fRRz]  "fRRz [N]"
  CPI tyre3/6 -> [mRRz]  "mRRz [Nm]"
  CPI tyre3/4 -> [mRRx]  "mRRx [Nm]"
  CPI tyre3/5 -> [mRRy]  "mRRy [Nm]"
  CPI tyre2/3 -> [fRLz]  "fRLz [N]"
  CPI tyre2/6 -> [mRLz]  "mRLz [Nm]"
  CPI tyre2/4 -> [mRLx]  "mRLx [Nm]"
  CPI tyre2/5 -> [mRLy]  "mRLy [Nm]"
  CPI tyre1/3 -> [fFRz]  "fFRz [N]"
  CPI tyre1/6 -> [mFRz]  "mFRz [Nm]"
  CPI tyre1/4 -> [mFRx]  "mFRx [Nm]"
  CPI tyre1/5 -> [mFRy]  "mFRy [Nm]"
  CPI tyre5/3 -> [fFLz]  "fFLz [N]"
  CPI tyre5/4 -> [mFLx]  "mFLx [Nm]"
  CPI tyre5/5 -> [mFLy]  "mFLy [Nm]"
  Bus Creator5/1 -> Tyre Mz Moments [Nm]/1
  [mFRz] -> Bus Creator5/2
  [mRLz] -> Bus Creator5/3
  [mRRz] -> Bus Creator5/4
  [mFLz] -> Bus Creator5/1
  [mFLy] -> Bus Creator4/1
  [mRRy] -> Bus Creator4/4
  [mRLy] -> Bus Creator4/3
  [mFRy] -> Bus Creator4/2
  Bus Creator4/1 -> Tyre My Moments [Nm]/1
  Bus Creator3/1 -> Tyre Mx Moments [Nm]/1
  [mFRx] -> Bus Creator3/2
  [mRLx] -> Bus Creator3/3
  [mRRx] -> Bus Creator3/4
  [mFLx] -> Bus Creator3/1
  [fFLz] -> Bus Creator2/1
  [fRRz] -> Bus Creator2/4
  [fRLz] -> Bus Creator2/3
  [fFRz] -> Bus Creator2/2
  Bus Creator2/1 -> Tyre z Forces [N]/1
  Bus Creator1/1 -> Tyre y Forces [N]/1
  Bus Creator/1 -> Tyre x Forces [N]/1
  [fFRy] -> Bus Creator1/2
  [fRLy] -> Bus Creator1/3
  [fRRy] -> Bus Creator1/4
  [fFLy] -> Bus Creator1/1
  [fRRx] -> Bus Creator/4
  [fRLx] -> Bus Creator/3
  [fFRx] -> Bus Creator/2
  [fFLx] -> Bus Creator/1
  CPI tyre3/2 -> [fRRy]  "fRRy [N]"
  CPI tyre2/2 -> [fRLy]  "fRLy [N]"
  CPI tyre1/2 -> [fFRy]  "fFRy [N]"
  CPI tyre5/2 -> [fFLy]  "fFLy [N]"
  CPI tyre2/1 -> [fRLx]  "fRLx [N]"
  CPI tyre3/1 -> [fRRx]  "fRRx [N]"
  CPI tyre1/1 -> [fFRx]  "fFRx [N]"
  CPI tyre5/1 -> [fFLx]  "fFLx [N]"
  CPI tyre3/7 -> Terminator18/1
  CPI tyre2/7 -> Terminator10/1
  CPI tyre1/7 -> Terminator9/1
  CPI tyre5/7 -> Terminator3/1
  CPI tyre5/6 -> [mFLz]  "mFLz [Nm]"
  VRRx [m/s]/1 -> CPI tyre3/2
  VRRy [m/s]/1 -> CPI tyre3/3
  VRLy [m/s]/1 -> CPI tyre2/3
  VRLx [m/s]/1 -> CPI tyre2/2
  VFRy [m/s]/1 -> CPI tyre1/3
  VFRx [m/s]/1 -> CPI tyre1/2
  VFLx [m/s]/1 -> CPI tyre5/2
  VFLy [m/s]/1 -> CPI tyre5/3
  omegaRR [rad/s]/1 -> CPI tyre3/1
  omegaRL [rad/s]/1 -> CPI tyre2/1
  omegaFR [rad/s]/1 -> CPI tyre1/1
  omegaFL [rad/s]/1 -> CPI tyre5/1
  Constant7/1 -> CPI tyre1/7
  Constant6/1 -> CPI tyre3/7
  Constant5/1 -> CPI tyre2/7
  Constant4/1 -> CPI tyre5/7
  Constant3/1 -> CPI tyre3/5
  Constant2/1 -> CPI tyre2/5
  Constant1/1 -> CPI tyre1/5
  Constant/1 -> CPI tyre5/5
  fFLz [N]/1 -> CPI tyre5/6
  fRLz [N]/1 -> CPI tyre2/6
  fRRz [N]/1 -> CPI tyre3/6
  fFRz [N]/1 -> CPI tyre1/6

== system VDSE_2019b/14-DOF VEHICLE MODEL/WHEEL ASSEMBLY/WHEEL ASSEMBLY PACEIJKA/SIDE SLIP ANGLE CALCULATION ==
  Vx [m/s] : Inport
  Vy [m/s] : Inport  Port=2
  Add : Sum
  Atan2 : Trigonometry  Operator=atan2
  Clock : Clock
  Constant : Constant  Value=enableLongDynamics
  Constant1 : Constant  Value=Vx0
  Constant2 : Constant  Value=0
  Sqrt : Sqrt
  Square : Math  Operator=square
  Square1 : Math  Operator=square
  Switch : Switch  Criteria=u2 > Threshold  SaturateOnIntegerOverflow=off  InputSameDT=off
  Switch1 : Switch  Criteria=u2 > Threshold  Threshold=0.01  SaturateOnIntegerOverflow=off  InputSameDT=off
  Vy [m/s]1 : InportShadow  Port=2
  V [m/s] : Outport
  beta [rad] : Outport  Port=2
  wires:
  Vy [m/s]1/1 -> Atan2/1
  Atan2/1 -> beta [rad]/1
  Sqrt/1 -> V [m/s]/1
  Add/1 -> Sqrt/1
  Vx [m/s]/1 -> Switch/1
  Vy [m/s]/1 -> Square1/1
  Square/1 -> Add/1
  Square1/1 -> Add/2
  Switch/1 -> Atan2/2, Square/1
  Constant/1 -> Switch1/1
  Constant1/1 -> Switch/3
  Switch1/1 -> Switch/2
  Constant2/1 -> Switch1/3
  Clock/1 -> Switch1/2

== system VDSE_2019b/14-DOF VEHICLE MODEL/WHEEL ASSEMBLY/WHEEL ASSEMBLY PACEIJKA/TIRE PARAMETERS ==
  Mux1 : Mux  Inputs=91
  Mux2 : Mux  Inputs=91
  TIRE PARAMETERS - FRONT AXLE : Subsystem
  TIRE PARAMETERS - REAR AXLE : Subsystem
  Tire Parameters Front Axle : Outport
  Tire Parameters Rear Axle : Outport  Port=2
  wires:
  TIRE PARAMETERS - FRONT AXLE/29(PCY1) -> Mux1/29
  TIRE PARAMETERS - FRONT AXLE/18(PKY3) -> Mux1/18
  TIRE PARAMETERS - FRONT AXLE/1(PHX1) -> Mux1/1
  TIRE PARAMETERS - FRONT AXLE/48(RVY4) -> Mux1/48
  TIRE PARAMETERS - FRONT AXLE/41(RBY1) -> Mux1/41
  TIRE PARAMETERS - FRONT AXLE/8(PEX3) -> Mux1/8
  TIRE PARAMETERS - FRONT AXLE/23(PHY1) -> Mux1/23
  TIRE PARAMETERS - FRONT AXLE/46(RVY2) -> Mux1/46
  TIRE PARAMETERS - FRONT AXLE/5(PCX1) -> Mux1/5
  TIRE PARAMETERS - FRONT AXLE/19(PVY1) -> Mux1/19
  TIRE PARAMETERS - FRONT AXLE/22(PVY4) -> Mux1/22
  TIRE PARAMETERS - FRONT AXLE/53(RHY1) -> Mux1/53
  TIRE PARAMETERS - FRONT AXLE/7(PEX2) -> Mux1/7
  TIRE PARAMETERS - FRONT AXLE/37(RCX1) -> Mux1/37
  TIRE PARAMETERS - FRONT AXLE/51(REY1) -> Mux1/51
  TIRE PARAMETERS - FRONT AXLE/28(PDY3) -> Mux1/28
  TIRE PARAMETERS - FRONT AXLE/36(RBX2) -> Mux1/36
  TIRE PARAMETERS - FRONT AXLE/34(ey) -> Mux1/34
  TIRE PARAMETERS - FRONT AXLE/10(PKX1) -> Mux1/10
  TIRE PARAMETERS - FRONT AXLE/30(PEY1) -> Mux1/30
  TIRE PARAMETERS - FRONT AXLE/17(PKY2) -> Mux1/17
  TIRE PARAMETERS - FRONT AXLE/2(PHX2) -> Mux1/2
  TIRE PARAMETERS - FRONT AXLE/33(PEY4) -> Mux1/33
  TIRE PARAMETERS - FRONT AXLE/39(REX2) -> Mux1/39
  TIRE PARAMETERS - FRONT AXLE/45(RVY1) -> Mux1/45
  TIRE PARAMETERS - FRONT AXLE/52(REY2) -> Mux1/52
  TIRE PARAMETERS - FRONT AXLE/21(PVY3) -> Mux1/21
  TIRE PARAMETERS - FRONT AXLE/3(PDX1) -> Mux1/3
  TIRE PARAMETERS - FRONT AXLE/6(PEX1) -> Mux1/6
  TIRE PARAMETERS - FRONT AXLE/4(PDX2) -> Mux1/4
  TIRE PARAMETERS - FRONT AXLE/49(RVY5) -> Mux1/49
  TIRE PARAMETERS - FRONT AXLE/44(RCY1) -> Mux1/44
  TIRE PARAMETERS - FRONT AXLE/25(PHY3) -> Mux1/25
  TIRE PARAMETERS - FRONT AXLE/24(PHY2) -> Mux1/24
  TIRE PARAMETERS - FRONT AXLE/54(RHY2) -> Mux1/54
  TIRE PARAMETERS - FRONT AXLE/43(RBY3) -> Mux1/43
  TIRE PARAMETERS - FRONT AXLE/13(ex) -> Mux1/13
  TIRE PARAMETERS - FRONT AXLE/31(PEY2) -> Mux1/31
  TIRE PARAMETERS - FRONT AXLE/14(PVX1) -> Mux1/14
  TIRE PARAMETERS - FRONT AXLE/35(RBX1) -> Mux1/35
  TIRE PARAMETERS - FRONT AXLE/15(PVX2) -> Mux1/15
  TIRE PARAMETERS - FRONT AXLE/27(PDY2) -> Mux1/27
  TIRE PARAMETERS - FRONT AXLE/20(PVY2) -> Mux1/20
  TIRE PARAMETERS - FRONT AXLE/11(PKX2) -> Mux1/11
  TIRE PARAMETERS - FRONT AXLE/50(RVY6) -> Mux1/50
  TIRE PARAMETERS - FRONT AXLE/32(PEY3) -> Mux1/32
  Mux1/1 -> Tire Parameters Front Axle/1
  TIRE PARAMETERS - FRONT AXLE/47(RVY3) -> Mux1/47
  TIRE PARAMETERS - FRONT AXLE/9(PEX4) -> Mux1/9
  TIRE PARAMETERS - FRONT AXLE/40(RHX1) -> Mux1/40
  TIRE PARAMETERS - FRONT AXLE/38(REX1) -> Mux1/38
  TIRE PARAMETERS - FRONT AXLE/42(RBY2) -> Mux1/42
  TIRE PARAMETERS - FRONT AXLE/26(PDY1) -> Mux1/26
  TIRE PARAMETERS - FRONT AXLE/12(PKX3) -> Mux1/12
  TIRE PARAMETERS - FRONT AXLE/16(PKY1) -> Mux1/16
  TIRE PARAMETERS - REAR AXLE/16(PKY1) -> Mux2/16
  TIRE PARAMETERS - REAR AXLE/12(PKX3) -> Mux2/12
  TIRE PARAMETERS - REAR AXLE/26(PDY1) -> Mux2/26
  TIRE PARAMETERS - REAR AXLE/42(RBY2) -> Mux2/42
  TIRE PARAMETERS - REAR AXLE/38(REX1) -> Mux2/38
  TIRE PARAMETERS - REAR AXLE/40(RHX1) -> Mux2/40
  TIRE PARAMETERS - REAR AXLE/9(PEX4) -> Mux2/9
  TIRE PARAMETERS - REAR AXLE/47(RVY3) -> Mux2/47
  Mux2/1 -> Tire Parameters Rear Axle/1
  TIRE PARAMETERS - REAR AXLE/32(PEY3) -> Mux2/32
  TIRE PARAMETERS - REAR AXLE/50(RVY6) -> Mux2/50
  TIRE PARAMETERS - REAR AXLE/11(PKX2) -> Mux2/11
  TIRE PARAMETERS - REAR AXLE/20(PVY2) -> Mux2/20
  TIRE PARAMETERS - REAR AXLE/27(PDY2) -> Mux2/27
  TIRE PARAMETERS - REAR AXLE/15(PVX2) -> Mux2/15
  TIRE PARAMETERS - REAR AXLE/35(RBX1) -> Mux2/35
  TIRE PARAMETERS - REAR AXLE/14(PVX1) -> Mux2/14
  TIRE PARAMETERS - REAR AXLE/31(PEY2) -> Mux2/31
  TIRE PARAMETERS - REAR AXLE/13(ex) -> Mux2/13
  TIRE PARAMETERS - REAR AXLE/43(RBY3) -> Mux2/43
  TIRE PARAMETERS - REAR AXLE/54(RHY2) -> Mux2/54
  TIRE PARAMETERS - REAR AXLE/24(PHY2) -> Mux2/24
  TIRE PARAMETERS - REAR AXLE/25(PHY3) -> Mux2/25
  TIRE PARAMETERS - REAR AXLE/44(RCY1) -> Mux2/44
  TIRE PARAMETERS - REAR AXLE/49(RVY5) -> Mux2/49
  TIRE PARAMETERS - REAR AXLE/4(PDX2) -> Mux2/4
  TIRE PARAMETERS - REAR AXLE/6(PEX1) -> Mux2/6
  TIRE PARAMETERS - REAR AXLE/3(PDX1) -> Mux2/3
  TIRE PARAMETERS - REAR AXLE/21(PVY3) -> Mux2/21
  TIRE PARAMETERS - REAR AXLE/52(REY2) -> Mux2/52
  TIRE PARAMETERS - REAR AXLE/45(RVY1) -> Mux2/45
  TIRE PARAMETERS - REAR AXLE/39(REX2) -> Mux2/39
  TIRE PARAMETERS - REAR AXLE/33(PEY4) -> Mux2/33
  TIRE PARAMETERS - REAR AXLE/2(PHX2) -> Mux2/2
  TIRE PARAMETERS - REAR AXLE/17(PKY2) -> Mux2/17
  TIRE PARAMETERS - REAR AXLE/30(PEY1) -> Mux2/30
  TIRE PARAMETERS - REAR AXLE/10(PKX1) -> Mux2/10
  TIRE PARAMETERS - REAR AXLE/34(ey) -> Mux2/34
  TIRE PARAMETERS - REAR AXLE/36(RBX2) -> Mux2/36
  TIRE PARAMETERS - REAR AXLE/28(PDY3) -> Mux2/28
  TIRE PARAMETERS - REAR AXLE/51(REY1) -> Mux2/51
  TIRE PARAMETERS - REAR AXLE/37(RCX1) -> Mux2/37
  TIRE PARAMETERS - REAR AXLE/7(PEX2) -> Mux2/7
  TIRE PARAMETERS - REAR AXLE/53(RHY1) -> Mux2/53
  TIRE PARAMETERS - REAR AXLE/22(PVY4) -> Mux2/22
  TIRE PARAMETERS - REAR AXLE/19(PVY1) -> Mux2/19
  TIRE PARAMETERS - REAR AXLE/5(PCX1) -> Mux2/5
  TIRE PARAMETERS - REAR AXLE/46(RVY2) -> Mux2/46
  TIRE PARAMETERS - REAR AXLE/23(PHY1) -> Mux2/23
  TIRE PARAMETERS - REAR AXLE/8(PEX3) -> Mux2/8
  TIRE PARAMETERS - REAR AXLE/41(RBY1) -> Mux2/41
  TIRE PARAMETERS - REAR AXLE/48(RVY4) -> Mux2/48
  TIRE PARAMETERS - REAR AXLE/1(PHX1) -> Mux2/1
  TIRE PARAMETERS - REAR AXLE/18(PKY3) -> Mux2/18
  TIRE PARAMETERS - REAR AXLE/29(PCY1) -> Mux2/29
  TIRE PARAMETERS - REAR AXLE/55(FNOMIN) -> Mux2/55
  TIRE PARAMETERS - FRONT AXLE/55(FNOMIN) -> Mux1/55
  TIRE PARAMETERS - FRONT AXLE/56(QHZ1) -> Mux1/56
  TIRE PARAMETERS - FRONT AXLE/57(QHZ2) -> Mux1/57
  TIRE PARAMETERS - FRONT AXLE/58(QHZ3) -> Mux1/58
  TIRE PARAMETERS - FRONT AXLE/59(QHZ4) -> Mux1/59
  TIRE PARAMETERS - FRONT AXLE/60(QBZ1) -> Mux1/60
  TIRE PARAMETERS - FRONT AXLE/61(QBZ2) -> Mux1/61
  TIRE PARAMETERS - FRONT AXLE/62(QBZ3) -> Mux1/62
  TIRE PARAMETERS - FRONT AXLE/63(QBZ4) -> Mux1/63
  TIRE PARAMETERS - FRONT AXLE/64(QBZ5) -> Mux1/64
  TIRE PARAMETERS - FRONT AXLE/65(QCZ1) -> Mux1/65
  TIRE PARAMETERS - FRONT AXLE/66(QDZ1) -> Mux1/66
  TIRE PARAMETERS - FRONT AXLE/67(QDZ2) -> Mux1/67
  TIRE PARAMETERS - FRONT AXLE/68(QDZ3) -> Mux1/68
  TIRE PARAMETERS - FRONT AXLE/69(QDZ4) -> Mux1/69
  TIRE PARAMETERS - FRONT AXLE/70(QEZ1) -> Mux1/70
  TIRE PARAMETERS - FRONT AXLE/71(QEZ2) -> Mux1/71
  TIRE PARAMETERS - FRONT AXLE/72(QEZ3) -> Mux1/72
  TIRE PARAMETERS - FRONT AXLE/73(QEZ4) -> Mux1/73
  TIRE PARAMETERS - FRONT AXLE/74(QEZ5) -> Mux1/74
  TIRE PARAMETERS - FRONT AXLE/75(QBZ9) -> Mux1/75
  TIRE PARAMETERS - FRONT AXLE/76(QBZ10) -> Mux1/76
  TIRE PARAMETERS - FRONT AXLE/77(QDZ6) -> Mux1/77
  TIRE PARAMETERS - FRONT AXLE/78(QDZ7) -> Mux1/78
  TIRE PARAMETERS - FRONT AXLE/79(QDZ8) -> Mux1/79
  TIRE PARAMETERS - FRONT AXLE/80(QDZ9) -> Mux1/80
  TIRE PARAMETERS - FRONT AXLE/81(R0) -> Mux1/81
  TIRE PARAMETERS - FRONT AXLE/82(zeta7) -> Mux1/82
  TIRE PARAMETERS - FRONT AXLE/83(SSZ1) -> Mux1/83
  TIRE PARAMETERS - FRONT AXLE/84(SSZ2) -> Mux1/84
  TIRE PARAMETERS - FRONT AXLE/85(SSZ3) -> Mux1/85
  TIRE PARAMETERS - FRONT AXLE/86(SSZ4) -> Mux1/86
  TIRE PARAMETERS - FRONT AXLE/87(QSY1) -> Mux1/87
  TIRE PARAMETERS - FRONT AXLE/88(QSY2) -> Mux1/88
  TIRE PARAMETERS - FRONT AXLE/89(QSY3) -> Mux1/89
  TIRE PARAMETERS - FRONT AXLE/90(QSY4) -> Mux1/90
  TIRE PARAMETERS - FRONT AXLE/91(VREF) -> Mux1/91
  TIRE PARAMETERS - REAR AXLE/56(QHZ1) -> Mux2/56
  TIRE PARAMETERS - REAR AXLE/57(QHZ2) -> Mux2/57
  TIRE PARAMETERS - REAR AXLE/58(QHZ3) -> Mux2/58
  TIRE PARAMETERS - REAR AXLE/59(QHZ4) -> Mux2/59
  TIRE PARAMETERS - REAR AXLE/60(QBZ1) -> Mux2/60
  TIRE PARAMETERS - REAR AXLE/61(QBZ2) -> Mux2/61
  TIRE PARAMETERS - REAR AXLE/62(QBZ3) -> Mux2/62
  TIRE PARAMETERS - REAR AXLE/63(QBZ4) -> Mux2/63
  TIRE PARAMETERS - REAR AXLE/64(QBZ5) -> Mux2/64
  TIRE PARAMETERS - REAR AXLE/65(QCZ1) -> Mux2/65
  TIRE PARAMETERS - REAR AXLE/66(QDZ1) -> Mux2/66
  TIRE PARAMETERS - REAR AXLE/67(QDZ2) -> Mux2/67
  TIRE PARAMETERS - REAR AXLE/68(QDZ3) -> Mux2/68
  TIRE PARAMETERS - REAR AXLE/69(QDZ4) -> Mux2/69
  TIRE PARAMETERS - REAR AXLE/70(QEZ1) -> Mux2/70
  TIRE PARAMETERS - REAR AXLE/71(QEZ2) -> Mux2/71
  TIRE PARAMETERS - REAR AXLE/72(QEZ3) -> Mux2/72
  TIRE PARAMETERS - REAR AXLE/73(QEZ4) -> Mux2/73
  TIRE PARAMETERS - REAR AXLE/74(QEZ5) -> Mux2/74
  TIRE PARAMETERS - REAR AXLE/75(QBZ9) -> Mux2/75
  TIRE PARAMETERS - REAR AXLE/76(QBZ10) -> Mux2/76
  TIRE PARAMETERS - REAR AXLE/77(QDZ6) -> Mux2/77
  TIRE PARAMETERS - REAR AXLE/78(QDZ7) -> Mux2/78
  TIRE PARAMETERS - REAR AXLE/79(QDZ8) -> Mux2/79
  TIRE PARAMETERS - REAR AXLE/80(QDZ9) -> Mux2/80
  TIRE PARAMETERS - REAR AXLE/81(R0) -> Mux2/81
  TIRE PARAMETERS - REAR AXLE/82(zeta7) -> Mux2/82
  TIRE PARAMETERS - REAR AXLE/83(SSZ1) -> Mux2/83
  TIRE PARAMETERS - REAR AXLE/84(SSZ2) -> Mux2/84
  TIRE PARAMETERS - REAR AXLE/85(SSZ3) -> Mux2/85
  TIRE PARAMETERS - REAR AXLE/86(SSZ4) -> Mux2/86
  TIRE PARAMETERS - REAR AXLE/87(QSY1) -> Mux2/87
  TIRE PARAMETERS - REAR AXLE/88(QSY2) -> Mux2/88
  TIRE PARAMETERS - REAR AXLE/89(QSY3) -> Mux2/89
  TIRE PARAMETERS - REAR AXLE/90(QSY4) -> Mux2/90
  TIRE PARAMETERS - REAR AXLE/91(VREF) -> Mux2/91

== system VDSE_2019b/14-DOF VEHICLE MODEL/SUSPENSION/FRONT SUSPENSION/SUSPENSION FL/FL ==
  z [m] : Inport
  Vz [m/s] : Inport  Port=2
  phi [rad] : Inport  Port=3
  phi_dot [rad/s] : Inport  Port=4
  theta [rad] : Inport  Port=5
  theta_dot [rad/s] : Inport  Port=6
  zFR [m] : Inport  Port=7
  yFL_road [m] : Inport  Port=8
  Constant : Constant  Value=zFL_dot0
  Constant1 : Constant  Value=zFL0
  Constant10 : Constant  Value=ctF
  Constant2 : Constant  Value=cF
  Constant3 : Constant  Value=wF
  Constant4 : Constant  Value=lF
  Constant5 : Constant  Value=kF
  Constant6 : Constant  Value=kRF
  Constant7 : Constant  Value=ktF
  Constant8 : Constant  Value=mF
  Constant9 : Constant  Value=g
  Derivative : Derivative
  Integrator : Integrator  InitialConditionSource=external
  Integrator1 : Integrator  InitialConditionSource=external
  MATLAB Function : MATLAB Function  TreatAsAtomicUnit=on
  zFL [m] : Outport
  zFL_dot [m/s] : Outport  Port=2
  wires:
  Constant9/1 -> MATLAB Function/9(g)
  Constant8/1 -> MATLAB Function/1(mF)
  Constant7/1 -> MATLAB Function/5(ktF)
  Constant6/1 -> MATLAB Function/4(kRF)
  Constant5/1 -> MATLAB Function/3(kF)
  Constant4/1 -> MATLAB Function/8(lF)
  Constant3/1 -> MATLAB Function/7(wF)
  Constant2/1 -> MATLAB Function/2(cF)
  zFR [m]/1 -> MATLAB Function/18(zFR)
  theta_dot [rad/s]/1 -> MATLAB Function/17(theta_dot)
  theta [rad]/1 -> MATLAB Function/16(theta)
  phi [rad]/1 -> MATLAB Function/14(phi)
  z [m]/1 -> MATLAB Function/12(z)
  yFL_road [m]/1 -> Derivative/1, MATLAB Function/10(yFL_road)
  Integrator/1 -> zFL [m]/1, MATLAB Function/19(zFL)  "zFL"
  Integrator1/1 -> zFL_dot [m/s]/1, MATLAB Function/20(zFL_dot), Integrator/1  "zFL_dot"
  MATLAB Function/1(zFL_dot_dot) -> Integrator1/1  "zFL_dot_dot"
  Vz [m/s]/1 -> MATLAB Function/13(Vz)
  phi_dot [rad/s]/1 -> MATLAB Function/15(phi_dot)
  Constant/1 -> Integrator1/2
  Constant1/1 -> Integrator/2
  Constant10/1 -> MATLAB Function/6(ctF)
  Derivative/1 -> MATLAB Function/11(yFL_road_dot)

== system VDSE_2019b/14-DOF VEHICLE MODEL/SUSPENSION/FRONT SUSPENSION/SUSPENSION FL/TIRE VERTICAL DEFLECTION ==
  zFL [m] : Inport
  zFL_dot [m/s] : Inport  Port=2
  yFL_road [m] : Inport  Port=3
  Add : Sum  Inputs=+-
  Add1 : Sum  Inputs=+-
  Add2 : Sum
  Derivative : Derivative
  Gain : Gain  Gain=-ktF
  Gain1 : Gain  Gain=-ctF
  yFL_road [m]1 : InportShadow  Port=3
  fFLz [N] : Outport
  wires:
  yFL_road [m]/1 -> Add/2
  zFL [m]/1 -> Add/1
  Add/1 -> Gain/1  "tire deflection FL"
  Gain/1 -> Add2/1
  yFL_road [m]1/1 -> Derivative/1
  Derivative/1 -> Add1/2
  zFL_dot [m/s]/1 -> Add1/1
  Add1/1 -> Gain1/1  "tire vertical velocity FL"
  Gain1/1 -> Add2/2
  Add2/1 -> fFLz [N]/1

== system VDSE_2019b/14-DOF VEHICLE MODEL/SUSPENSION/FRONT SUSPENSION/SUSPENSION FR/FR ==
  z [m] : Inport
  Vz [m/s] : Inport  Port=2
  phi [rad] : Inport  Port=3
  phi_dot [rad/s] : Inport  Port=4
  theta [rad] : Inport  Port=5
  theta_dot [rad/s] : Inport  Port=6
  zFL [m] : Inport  Port=7
  yFR_road [m] : Inport  Port=8
  Constant : Constant  Value=zFR_dot0
  Constant1 : Constant  Value=zFR0
  Constant10 : Constant  Value=ctF
  Constant2 : Constant  Value=cF
  Constant3 : Constant  Value=wF
  Constant4 : Constant  Value=lF
  Constant5 : Constant  Value=kF
  Constant6 : Constant  Value=kRF
  Constant7 : Constant  Value=ktF
  Constant8 : Constant  Value=mF
  Constant9 : Constant  Value=g
  Derivative : Derivative
  Integrator : Integrator  InitialConditionSource=external
  Integrator1 : Integrator  InitialConditionSource=external
  MATLAB Function : MATLAB Function  TreatAsAtomicUnit=on
  zFR [m] : Outport
  zFR_dot [m/s] : Outport  Port=2
  wires:
  Constant9/1 -> MATLAB Function/9(g)
  Constant8/1 -> MATLAB Function/1(mF)
  Constant7/1 -> MATLAB Function/8(ktF)
  Constant6/1 -> MATLAB Function/6(kRF)
  Constant5/1 -> MATLAB Function/5(kF)
  Constant4/1 -> MATLAB Function/4(lF)
  Constant3/1 -> MATLAB Function/3(wF)
  Constant2/1 -> MATLAB Function/2(cF)
  zFL [m]/1 -> MATLAB Function/18(zFL)
  theta_dot [rad/s]/1 -> MATLAB Function/17(theta_dot)
  theta [rad]/1 -> MATLAB Function/16(theta)
  phi_dot [rad/s]/1 -> MATLAB Function/15(phi_dot)
  phi [rad]/1 -> MATLAB Function/14(phi)
  Vz [m/s]/1 -> MATLAB Function/13(Vz)
  yFR_road [m]/1 -> Derivative/1, MATLAB Function/10(yFR_road)
  Integrator/1 -> zFR [m]/1, MATLAB Function/19(zFR)  "zFR"
  Integrator1/1 -> MATLAB Function/20(zFR_dot), zFR_dot [m/s]/1, Integrator/1  "zFR_dot"
  MATLAB Function/1(zFR_dot_dot) -> Integrator1/1  "zFR_dot_dot"
  z [m]/1 -> MATLAB Function/12(z)
  Constant/1 -> Integrator1/2
  Constant1/1 -> Integrator/2
  Constant10/1 -> MATLAB Function/7(ctF)
  Derivative/1 -> MATLAB Function/11(yFR_road_dot)

== system VDSE_2019b/14-DOF VEHICLE MODEL/SUSPENSION/FRONT SUSPENSION/SUSPENSION FR/TIRE VERTICAL DEFLECTION ==
  zFR [m] : Inport
  zFR_dot [m/s] : Inport  Port=2
  yFR_road [m] : Inport  Port=3
  Add : Sum  Inputs=+-
  Add1 : Sum
  Add2 : Sum  Inputs=+-
  Derivative : Derivative
  Gain : Gain  Gain=-ktF
  Gain1 : Gain  Gain=-ctF
  yFR_road [m]1 : InportShadow  Port=3
  fFRz [N] : Outport
  wires:
  yFR_road [m]/1 -> Add/2
  zFR [m]/1 -> Add/1
  Add/1 -> Gain/1  "tire deflection FR"
  Gain/1 -> Add1/1
  yFR_road [m]1/1 -> Derivative/1
  Derivative/1 -> Add2/2
  zFR_dot [m/s]/1 -> Add2/1
  Add2/1 -> Gain1/1  "tire vertical velocity FR"
  Gain1/1 -> Add1/2
  Add1/1 -> fFRz [N]/1
